simulink model "CarTempSensor"  (R2020b)
settings: Solver=VariableStepAuto  StartTime=0.0  StopTime=10.0  RelTol=1e-3
settings Model: Creator=99003747  LastModifiedBy=99003747

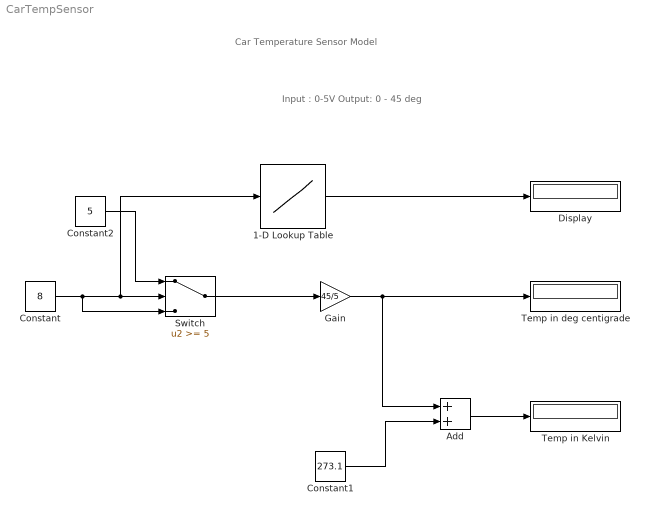
== system CarTempSensor ==
  note: Input : 0-5V
      | Output: 0 - 45 deg
  note: Car Temperature Sensor Model
  1-D Lookup Table : Lookup_n-D  NumberOfTableDimensions=1  BreakpointsForDimension1=[0:1:5]  Table=[0:9:45]  InternalRulePriority=Speed  RndMeth=Simplest  InputSameDT=on
  Add : Sum
  Constant : Constant  Value=8
  Constant1 : Constant  Value=273.1
  Constant2 : Constant  Value=5
  Display : Display
  Gain : Gain  Gain=45/5
  Switch : Switch  Threshold=5
  Temp in Kelvin : Display
  Temp in deg centigrade : Display
  wires:
  Gain/1 -> Add/1, Temp in deg centigrade/1
  Constant1/1 -> Add/2
  Add/1 -> Temp in Kelvin/1
  Constant/1 -> 1-D Lookup Table/1, Switch/2, Switch/3
  Switch/1 -> Gain/1
  Constant2/1 -> Switch/1
  1-D Lookup Table/1 -> Display/1
